simulink model "HrmncDrv"  (R2019a)
settings: Solver=VariableStepAuto  StartTime=0.0  StopTime=10.0  RelTol=1e-3
undefined symbols (not defined in the file or in its folder): N
libraries: simulink x2
settings Model: DataDictionary=HrmncDrv.sldd  Creator=chiha  LastModifiedBy=chiha

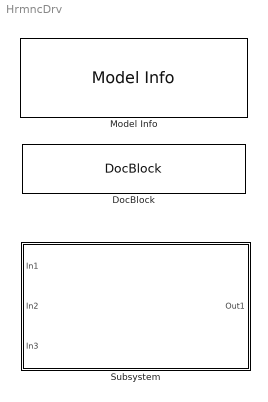
== system HrmncDrv ==
  DocBlock : simulink/Model-Wide Utilities/DocBlock  DocumentType=Text
      content=|
      | Type your documentation here
  Model Info : simulink/Model-Wide Utilities/Model Info  Frame=on  DisplayStringWithTags=|  HorizontalTextAlignment=Center  LeftAlignmentValue=0.5
      | Model Info
      | %<ModelName>
      | %<Description>
      | %<LastModificationDate>
  Subsystem : Subsystem  TreatAsAtomicUnit=on
      settings: RTWSystemCode=Nonreusable function

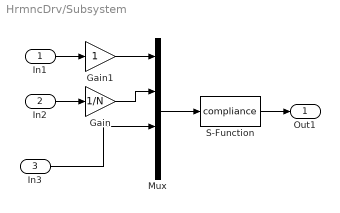
== system HrmncDrv/Subsystem ==
  In1 : Inport
  In2 : Inport  Port=2
  In3 : Inport  Port=3
  Gain : Gain  Gain=1/N
  Gain1 : Gain
  Mux : Mux
  S-Function : S-Function  FunctionName=compliance  SFunctionDeploymentMode=off  EnableBusSupport=off
  Out1 : Outport
  wires:
  S-Function/1 -> Out1/1
  Mux/1 -> S-Function/1
  Gain1/1 -> Mux/1
  In1/1 -> Gain1/1
  In2/1 -> Gain/1
  Gain/1 -> Mux/2
  In3/1 -> Mux/3
